simulink library "lib_affectiveChar_behavior"  (R2014a)
settings: Solver=ode45  StartTime=0.0  StopTime=10.0  RelTol=1e-3
libraries: simulink x5
(part 4 of 4)

== stateflow chart lib_affectiveChar_behavior/idlePoseRachel ==
  note: The higher BOREDOMT (treshold), the lower chance of bored pose.
  state stateRandomPose
    entry: interest=BOREDOM_THRESHOLD-boredom;
    entry: randPoseChance=randi([1,interest]);
  state sendBML(arg) [function]
  note: num of bmlID=18
  state stateBoredPose
    entry:
    sendBML( idlePoseRachelTable(randi([1,18])) );
  (default) -> stateRandomPose
  stateBoredPose -> stateRandomPose : after(1,secs)
  stateRandomPose -> (junction 2)
  (junction 2) -> stateRandomPose [order 2] : [randPoseChance~=1]
  (junction 2) -> stateRandomPose [order 3] : [isPosing~=0]
  (junction 2) -> stateBoredPose [order 1] : [([randPoseChance==1])&([isPosing==0])]
  data: arg function_input double size=[256 1]; bmlID function_input double; poseBML function_output double size=[256,1]; boredom data_store_memory size=2; BOREDOM_THRESHOLD data_store_memory size=2; randPoseChance data_store_memory size=2; isPosing data_store_memory size=2; interest data_store_memory size=2
  events: secs input RISING_EDGE_EVENT
  function poseBML=idlePoseRachelTable(bmlID):
    | function poseBML=idlePoseRachelTable(bmlID)
    | 
    | aVarTruthTableCondition_1 = false;
    | aVarTruthTableCondition_2 = false;
    | aVarTruthTableCondition_3 = false;
    | aVarTruthTableCondition_4 = false;
    | aVarTruthTableCondition_5 = false;
    | aVarTruthTableCondition_6 = false;
    | aVarTruthTableCondition_7 = false;
    | aVarTruthTableCondition_8 = false;
    | aVarTruthTableCondition_9 = false;
    | aVarTruthTableCondition_10 = false;
    | aVarTruthTableCondition_11 = false;
    | aVarTruthTableCondition_12 = false;
    | aVarTruthTableCondition_13 = false;
    | aVarTruthTableCondition_14 = false;
    | aVarTruthTableCondition_15 = false;
    | aVarTruthTableCondition_16 = false;
    | aVarTruthTableCondition_17 = false;
    | aVarTruthTableCondition_18 = false;
    | 
    | 
    | 
    | aVarTruthTableCondition_1 = logical(bmlID==1);
    | 
    | 
    | aVarTruthTableCondition_2 = logical(bmlID==2);
    | 
    | 
    | aVarTruthTableCondition_3 = logical(bmlID==3);
    | 
    | 
    | aVarTruthTableCondition_4 = logical(bmlID==4);
    | 
    | 
    | aVarTruthTableCondition_5 = logical(bmlID==5);
    | 
    | 
    | aVarTruthTableCondition_6 = logical(bmlID==6);
    | 
    | 
    | aVarTruthTableCondition_7 = logical(bmlID==7);
    | 
    | 
    | aVarTruthTableCondition_8 = logical(bmlID==8);
    | 
    | 
    | aVarTruthTableCondition_9 = logical(bmlID==9);
    | 
    | 
    | aVarTruthTableCondition_10 = logical(bmlID==10);
    | 
    | 
    | aVarTruthTableCondition_11 = logical(bmlID==11);
    | 
    | 
    | aVarTruthTableCondition_12 = logical(bmlID==12);
    | 
    | 
    | aVarTruthTableCondition_13 = logical(bmlID==13);
    | 
    | 
    | aVarTruthTableCondition_14 = logical(bmlID==14);
    | 
    | 
    | aVarTruthTableCondition_15 = logical(bmlID==15);
    | 
    | 
    | aVarTruthTableCondition_16 = logical(bmlID==16);
    | 
    | 
    | aVarTruthTableCondition_17 = logical(bmlID==17);
    | 
    | 
    | aVarTruthTableCondition_18 = logical(bmlID==18);
    | 
    | if (aVarTruthTableCondition_1)
    |     aFcnTruthTableAction_6();
    | elseif (aVarTruthTableCondition_2)
    |     aFcnTruthTableAction_2();
    | elseif (aVarTruthTableCondition_3)
    |     aFcnTruthTableAction_1();
    | elseif (aVarTruthTableCondition_4)
    |     aFcnTruthTableAction_2();
    | elseif (aVarTruthTableCondition_5)
    |     aFcnTruthTableAction_3();
    | elseif (aVarTruthTableCondition_6)
    |     aFcnTruthTableAction_7();
    | elseif (aVarTruthTableCondition_7)
    |     aFcnTruthTableAction_1();
    | elseif (aVarTruthTableCondition_8)
    |     aFcnTruthTableAction_3();
    | elseif (aVarTruthTableCondition_9)
    |     aFcnTruthTableAction_1();
    | elseif (aVarTruthTableCondition_10)
    |     aFcnTruthTableAction_6();
    | elseif (aVarTruthTableCondition_11)
    |     aFcnTruthTableAction_7();
    | elseif (aVarTruthTableCondition_12)
    |     aFcnTruthTableAction_5();
    | elseif (aVarTruthTableCondition_13)
    |     aFcnTruthTableAction_5();
    | elseif (aVarTruthTableCondition_14)
    |     aFcnTruthTableAction_3();
    | elseif (aVarTruthTableCondition_15)
    |     aFcnTruthTableAction_4();
    | elseif (aVarTruthTableCondition_16)
    |     aFcnTruthTableAction_3();
    | elseif (aVarTruthTableCondition_17)
    |     aFcnTruthTableAction_5();
    | elseif (aVarTruthTableCondition_18)
    |     aFcnTruthTableAction_5();
    | else % Default
    |     aFcnTruthTableAction_1();
    | end
    | 
    | function aFcnTruthTableAction_1()
    | 
    | % WeightShift
    | 
    | poseBML=encStr2Arr('<?xml version="1.0" ?><act><bml><animation name="ChrBrad@Idle01_WeightShift01" ready="1" relax="6" start="0" stroke="3 end="7"/></bml></act>');
    | 
    | function aFcnTruthTableAction_2()
    | 
    | % ScratchChest
    | 
    | poseBML=encStr2Arr('<?xml version="1.0" ?><act><bml><animation name="ChrRachel_ChrBrad@Idle01_ScratchChest01" /></bml></act>');
    | 
    | function aFcnTruthTableAction_3()
    | 
    | % ScratchHead
    | 
    | poseBML=encStr2Arr('<?xml version="1.0" ?><act><bml><animation name="ChrBrad@Idle01_ScratchHeadLf01" /></bml></act>');
    | 
    | function aFcnTruthTableAction_4()
    | 
    | % ShoulderStretchUpDown
    | 
    | poseBML=encStr2Arr('<?xml version="1.0" ?><act><bml><animation name="ChrBrad@Idle01_ShoulderStretch01" /></bml></act>');
    | 
    | function aFcnTruthTableAction_5()
    | 
    | % SqueezeHand01
    | 
    | poseBML=encStr2Arr('<?xml version="1.0" ?><act><bml><animation name="ChrBrad@Idle01_SqueezeHand01" /></bml></act>');
    | 
    | function aFcnTruthTableAction_6()
    | 
    | % WeightShift2
    | 
    | poseBML=encStr2Arr('<?xml version="1.0" ?><act><bml><animation name="ChrBrad@Idle01_WeightShift02" /></bml></act>');
    | 
    | function aFcnTruthTableAction_7()
    | 
    | % Idle01_ToIdle02
    | 
    | poseBML=encStr2Arr('<?xml version="1.0" ?><act><bml><animation name="ChrBrad@Idle01_ToIdle02" ready="1" relax="4" start="0" stroke="3" end="7"/></bml></act>');

== stateflow chart lib_affectiveChar_behavior/notImitateSmile ==
  state subSmile [parallel]
    settings: executionOrder=1
    state stateInitial
      entry: avert=1; gameState=14;
      n=encStr2Arr(' ');bmlsM=[n n n n n];newBmlsM=[n n n n n];
    state stateCheckSmile
    state gazeCamera
      entry:  [P,BMLM]= smileTable(2) ;avert=0;
      newBmlsM=insertQueue(bmlsM,BMLM);
      bmlsM=newBmlsM;
    state wait
    state checkP
      entry:  [P,BMLM]=  smileTable(1) ;
      newBmlsM=insertQueue(bmlsM,BMLM);
      bmlsM=newBmlsM;
    (default) -> stateInitial
    stateInitial -> stateCheckSmile
    subSmile.wait -> stateCheckSmile : after(10,secs)
    stateCheckSmile -> stateCheckSmile [order 2]
    gazeCamera -> stateCheckSmile [order 2] : after(1,secs)[isSmiling~=1]
    stateCheckSmile -> gazeCamera [order 1] : [[isSmiling==1]&[ gameState~= STATE_GO]&[ gameState~= STATE_READY]]
    checkP -> subSmile.wait
    gazeCamera -> checkP [order 1] : after(1,secs)[isSmiling==1]
  note: SMILE_DUER=10 seceonds
  note: check if still isSmiling is true works as a buffer to remove the smiles that last ony 1 sec (system errors).
  state subFacial [parallel]
    settings: executionOrder=2
    state stateFacialExpression
      entry:[au,au_L]=setAU(internalE);
      eAmountF =set_eAmountFactor(internalE,personality);
      BMLl=cmdBML_AUmerg(au,eAmountF);
      newBmlsL=insertQueueLow(bmlsL,BMLl);
      bmlsL=newBmlsL;
      %fprintf('%1.1f',internalE);disp(decArr2Str(BMLl));
    state initial
      entry:
      au=[0,0,0,0,0,0];
      au_L=0;
    state wait
    state wait2
    (default) -> initial
    subFacial.wait -> stateFacialExpression [order 1] : [internalE~=6]
    initial -> subFacial.wait
    stateFacialExpression -> subFacial.wait [order 1] : [internalE==6]
    subFacial.wait -> subFacial.wait [order 2]
    wait2 -> stateFacialExpression : [emoChange==1]
    stateFacialExpression -> wait2 [order 2] : [emoChange==0]
  data: bmls function_input double size=[1000,5]; myBML function_input double size=[1000,1]; newBmls function_output double size=[1000,5]; bmls function_input double size=[1000,5]; myBML function_input double size=[1000,1]; newBmls function_output double size=[1000,5]; bmlID function_input double; p function_output double size=1; poseBML function_output double size=[1000,1]; bmlID function_input double; p function_output double size=1; poseBML function_output double size=[1000,1]; E function_input double size=1; AU function_output double size=[1,6]; L function_output double size=1; E function_input double size=1; eAmountFactor function_output double size=[1,6]; Pt function_input double size=1; smileN local double size=1; isSmiling input double size=1 =0; avert data_store_memory =0; gazing data_store_memory size=2; GAZE_WIN data_store_memory size=2; BML data_store_memory size=[256,1]; P data_store_memory; fileID local double size=1; gameState output double; STATE_GO data_store_memory; STATE_READY data_store_memory; STATE_BEFORE data_store_memory; newBmlsM local double size=[1000,5]; bmlsM data_store_memory size=[256,1]; BMLM local double size=[1000,1]; n local; personality input double size=1; internalE input double size=1; au local; eAmountF local; emoChange input boolean size=1; au_i local double size=1; au_L local double size=1; emoDisp local; bmlsL data_store_memory size=[256,1]; BMLl local double size=[1000,1]; newBmlsL local double size=[1000,5]
  events: secs input RISING_EDGE_EVENT
  function newBmls =insertQueue(bmls,myBML):
    | function newBmls =insertQueue(bmls,myBML)
    |     full=1;
    |     t=encStr2Arr(' ');
    |     newBmls=[t t t t t];
    |     for i = 1:5
    |         if (isequal(bmls(:,i),t))
    |             %add to end of the queue where its empty
    |             bmls(:,i)=myBML;
    |             full=0;
    |             break
    |         end
    |     end
    |     if(full~=0)
    |             %if queue full, shift all elements to left which removes the first one, then add to end
    |             bmls(:,1)= bmls(:,2);
    |             bmls(:,2)= bmls(:,3);
    |             bmls(:,3)= bmls(:,4);
    |             bmls(:,5)=myBML;
    |     end
    |     newBmls=bmls;
  function newBmls =insertQueueLow(bmls,myBML):
    | function newBmls =insertQueueLow(bmls,myBML)
    |     full=1;
    |     t=encStr2Arr(' ');
    |     newBmls=[t t t t t];
    |     for i = 1:5
    |         if (isequal(bmls(:,i),t))
    |             %add to end of the queue where its empty
    |             bmls(:,i)=myBML;
    |             full=0;
    |             break
    |         end
    |     end
    |     if(full~=0)
    |             %if queue full, shift all elements to left which removes the first one, then add to end
    |             bmls(:,1)= bmls(:,2);
    |             bmls(:,2)= bmls(:,3);
    |             bmls(:,3)= bmls(:,4);
    |             bmls(:,5)=myBML;
    |     end
    |     newBmls=bmls;
  function [p,poseBML] = smileTable(bmlID):
    | function [p,poseBML] = smileTable(bmlID)
    | 
    | aVarTruthTableCondition_1 = false;
    | aVarTruthTableCondition_2 = false;
    | 
    | 
    | % smile
    | 
    | aVarTruthTableCondition_1 = logical(bmlID==1);
    | 
    | % headN
    | 
    | aVarTruthTableCondition_2 = logical(bmlID==2);
    | 
    | if (aVarTruthTableCondition_1)
    |     aFcnTruthTableAction_1();
    | elseif (aVarTruthTableCondition_2)
    |     aFcnTruthTableAction_2();
    | else % Default
    |     aFcnTruthTableAction_1();
    | end
    | 
    | function aFcnTruthTableAction_1()
    | 
    | % smile
    | 
    | poseBML=encStr2Arr('<?xml version="1.0"?><act><bml><face amount="1" au="12" side="BOTH" start="0" stroke="2" relax="3" end="4" type="facs"/><face amount="0.3" au="6" side="BOTH" start="0" stroke="2" relax="3" end="4" type="facs"/></bml></act>');p=3;
    | 
    | function aFcnTruthTableAction_2()
    | 
    | % headNeutralBrow
    | 
    | poseBML=encStr2Arr('<?xml version="1.0" ?><act><bml><gaze target="gazeTarget" start="0" end="5" sbm:time-hint="1.5"/></bml></act>');p=3;
    | 
    | function aFcnTruthTableAction_3()
    | 
    | % smileBrow
    | 
    | poseBML=encStr2Arr('<?xml version="1.0"?><act><bml><face amount="0.1" au="1" side="BOTH" start="0" stroke="2" relax="4" end="6" type="facs"/><face amount="0.1" au="2" side="BOTH" start="0" stroke="2" relax="4" end="6" type="facs"/></bml></act>');p=3;
  function [p,poseBML] = facialExpr(bmlID):
    | function [p,poseBML] = facialExpr(bmlID)
    | 
    | aVarTruthTableCondition_1 = false;
    | aVarTruthTableCondition_2 = false;
    | 
    | 
    | % smile
    | 
    | aVarTruthTableCondition_1 = logical(bmlID==1);
    | 
    | % headN
    | 
    | aVarTruthTableCondition_2 = logical(bmlID==2);
    | 
    | if (aVarTruthTableCondition_1)
    |     aFcnTruthTableAction_1();
    | elseif (aVarTruthTableCondition_2)
    |     aFcnTruthTableAction_2();
    | else % Default
    |     aFcnTruthTableAction_1();
    | end
    | 
    | function aFcnTruthTableAction_1()
    | 
    | % smile
    | 
    | poseBML=encStr2Arr('<?xml version="1.0"?><act><bml><face amount="1" au="12" side="BOTH" start="0" stroke="10" relax="70" end="100" type="facs"/><face amount="0.3" au="6" side="BOTH" start="0" stroke="10" relax="70" end="100" type="facs"/></bml></act>');p=3;
    | 
    | function aFcnTruthTableAction_2()
    | 
    | % headNeutralBrow
    | 
    | poseBML=encStr2Arr('<?xml version="1.0" ?><act><bml><gaze target="gazeTarget" start="0" end="5" sbm:time-hint="1.5"/></bml></act>');p=3;
    | 
    | function aFcnTruthTableAction_3()
    | 
    | % smileBrow
    | 
    | poseBML=encStr2Arr('<?xml version="1.0"?><act><bml><face amount="0.1" au="1" side="BOTH" start="0" stroke="2" relax="4" end="6" type="facs"/><face amount="0.1" au="2" side="BOTH" start="0" stroke="2" relax="4" end="6" type="facs"/></bml></act>');p=3;
  function [AU,L]=setAU(E):
    | function [AU,L]=setAU(E)	
    | % 1	Inner Brow Raiser,% 2	Outer Brow Raiser, % 4	Brow Lowerer
    | % 5	Upper Lid Raiser,% 6	Cheek Raiser,% 7	Lid Tightener
    | % 8	Lips Toward Each Other,% 9	Nose Wrinkler,% 10	Upper Lip Raiser	
    | % 11	Nasolabial Deepener	% 12	Lip Corner Puller % 13	Sharp Lip Puller % 14	Dimpler	
    | % 15	Lip Corner Depressor % 16	Lower Lip Depressor % 17	Chin Raiser	mentalis
    | % 18	Lip Pucker	% 19	Tongue Show	% 20	Lip Stretcher % 21	Neck Tightener	platysma
    | % 22	Lip Funneler% 23	Lip Tightener% 24	Lip Pressor % 25	Lips Part	depressor
    | % 26	Jaw Drop,% 27	Mouth Stretch
    | % 43	Eyes Closed, % 44	Eyebrow Gatherer,% 45	Blink,% 46	Wink
    | %smartbody no 43,15,17,10 looks wierd,no 142
    |    AU=[0,0,0,0,0,0];L=0;
    |    % AU5(eyeOpen) for A+
    |    % AU1,4 for V-
    |    %AU12 for V+
    |     switch(E)
    |         case 1 %V- A-,bored (43)[1]
    |             AU=[1,2,45,0,0,0];L=3;%[1,1,0.35]
    |         
    |         case 2 %V- A-;sad %(1,2,4,10,15,17,43)[];can be [1,2,4,45,6,0]
    |             AU=[1,4,0,0,0,0];L=2;%[1,1,0,0,0,0]
    |         
    |         case 3 %V- A+,frust(2,1,14)[1],(-1,-2,4,7,14)[2], maybe(1,7)[0.7,0.7,0.5]
    |             AU=[1,2,4,5,6,0];L=5;%[1,1,1,0.5,0.5,0]
    |         
    |         case 4 %V- A+,fear(1,2,4,5,25=mouth)
    |             AU=[1,2,4,5,6,7];L=6; %[1,1,1,0.2,0.2]
    |         
    |         case 5%V+ A-,calm
    |             AU=[12,14,0,0,0,0];L=2;%[0.7,0.3,0,0,0,0]
    |         
    |         case 7%V+ A+,happy
    |             AU=[6,12,0,0,0,0];L=2;%[1,0.5,0,0,0,0]
    |         
    |         case 8%V+ A+,excited
    |             AU=[12,26,5,1,2,0];L=5;%[1,1,1,1,1,0]
    |         
    |         case 9%V- A+, angry
    |             AU=[2,4,5,7,45,0];L=5;%[0.5,1,0.2,0.2,0.2]
    |         
    |         otherwise
    |             %confusion (1,2,4,7)[1] %[1,1,1,0.2]
    |             %worried (1,2,4,5) [1,1,1,0.5]
    |             %angry(4,5,7,10,27)[], can be(2,4,5,7,45)[0.5,1,0.2,0.2,0.2]
    | 
    |             AU=[0,0,0,0,0,0];L=0;
    |             disp('error, setAU,emotion not listed');
    |     end  
    | %[1]Craig S.D. et al(2004)emotions during learning:the first steps tw affect sensitive
    | %[2]grafsgard J F () automatically recog facial indicator of frust
  function eAmountFactor =set_eAmountFactor(E,Pt):
    | function eAmountFactor =set_eAmountFactor(E,Pt)
    |     AU=[0,0,0,0,0,0];eAmountFactor=[0,0,0,0,0,0];pFactor=0.5;
    |     %Note: make sure you change values in all 4 personalities
    |     if(Pt==1)
    |         %HEHN
    |         if(E==1)  %bored
    |             eAmountFactor=[1,1,0.37,0,0,0];
    |         elseif(E==2) %sad
    |             eAmountFactor=[1,1,0,0,0,0];
    |         elseif(E==3) %frust
    |             eAmountFactor=[1,1,1,0.5,0.5,0];
    |         elseif(E==4) %fear
    |             eAmountFactor=[1,1,1,0.2,0.2,0];
    |         elseif(E==5)%sleepy
    |             eAmountFactor=[0.7,0.3,0,0,0,0];
    |         elseif(E==7)%happy
    |             eAmountFactor=[0.38,1,0,0,0,0];
    |         elseif(E==8)%excited
    |             eAmountFactor=[0.5,0.2,0.6,0.6,0.6,0];    
    |         else          
    |             eAmountFactor=[0,0,0,0,0,0];
    |             disp('error, set_eAmountFactor,emotion not listed');
    |         end
    |     
    |         %LEHN  
    |     elseif(Pt==2)
    |         if(E==1)  %bored
    |             eAmountFactor=[1,1,0.37,0,0,0];
    |         elseif(E==2) %sad
    |             eAmountFactor=[1,1,0,0,0,0];
    |         elseif(E==3) %frust
    |             eAmountFactor=[1,1,1,0.5,0.5,0];
    |         elseif(E==4) %fear
    |             eAmountFactor=[1,1,1,0.2,0.2,0];
    |         elseif(E==5)%sleepy
    |             eAmountFactor=[0.7,0.3,0,0,0,0];
    |         elseif(E==7)%happy
    |             eAmountFactor=[0.38,1,0,0,0,0];
    |         elseif(E==8)%excited[12,26,5,1,2,0]
    |             eAmountFactor= [0.5,0.2,0.6,0.6,0.6,0];    
    |         else          
    |             eAmountFactor=[0,0,0,0,0,0];
    |             disp('error, set_eAmountFactor,emotion not listed');
    |         end
    | 
    |         %HELN
    |    elseif(Pt==3)
    |         if(E==1)  %bored
    |             eAmountFactor=[1,1,0.37,0,0,0];
    |         elseif(E==2) %sad
    |             eAmountFactor=[1,1,0,0,0,0];
    |         elseif(E==3) %frust
    |             eAmountFactor=[1,1,1,0.5,0.5,0];
    |         elseif(E==4) %fear
    |             eAmountFactor=[1,1,1,0.2,0.2,0];
    |         elseif(E==5)%sleepy
    |             eAmountFactor=[0.7,0.3,0,0,0,0];
    |         elseif(E==7)%happy
    |             eAmountFactor=[0.38,1,0,0,0,0];
    |         elseif(E==8)%excited[12,26,5,1,2,0]
    |             eAmountFactor=  [0.5,0.2,0.6,0.6,0.6,0];    
    |         else          
    |             eAmountFactor=[0,0,0,0,0,0];
    |             disp('error, set_eAmountFactor,emotion not listed');
    |         end
    |         eAmountFactor=eAmountFactor*pFactor;
    |         %LELN
    |     elseif(Pt==4)
    |         if(E==1)  %bored
    |             eAmountFactor=[1,1,0.37,0,0,0];
    |         elseif(E==2) %sad
    |             eAmountFactor=[1,1,0,0,0,0];
    |         elseif(E==3) %frust
    |             eAmountFactor=[1,1,1,0.5,0.5,0];
    |         elseif(E==4) %fear
    |             eAmountFactor=[1,1,1,0.2,0.2,0];
    |         elseif(E==5)%sleepy
    |             eAmountFactor=[0.7,0.3,0,0,0,0];
    |         elseif(E==7)%happy
    |             eAmountFactor=[0.38,1,0,0,0,0];
    |         elseif(E==8)%excited[12,26,5,1,2,0]
    |             eAmountFactor=  [0.5,0.2,0.6,0.6,0.6,0];    
    |         else          
    |             eAmountFactor=[0,0,0,0,0,0];
    |             disp('error, set_eAmountFactor,emotion not listed');
    |         end
    |         eAmountFactor=eAmountFactor*pFactor;
    |     end
    | %Following is if we want a same factor for each personaliy all through AUs
    | % function eAmountFactor =set_eAmountFactor(E,P)
    | %     AU=[6,12,142,0,0,0];eAMOUNT=[0,0,0,0,0,0];
    | %     switch E
    | %         case 1  %bored
    | %             eAMOUNT=[1,1,1,0,0,0];
    | %         case 2 %sad
    | %             eAMOUNT=[0.7,0.4,0.9,0,0,0];
    | %         case 3 %angry
    | %             eAMOUNT=[1,0.8,1,0,0,0];
    | %         case 4 %fear
    | %             eAMOUNT=[1,1,1,0,0,0];%5,6,7,26
    | %         case 5%contempt
    | %             eAMOUNT=[1,1,1,0,0,0];
    | %         case 7%happy
    | %             eAMOUNT=[0.2,1,0,0,0,0];
    | %         otherwise           
    | %             eAMOUNT=[0,0,0,0,0,0];
    | %             disp('error,amount for emotion not listed:');disp('eAMOUNT');
    | %     end 
    | %     switch P
    | %         case 1 %HEHN
    | %             pFactor=1;
    | %         case 2 %LEHN
    | %             pFactor=1;
    | %         case 3 %HELN
    | %             pFactor=0.5;
    | %         case 4 %LELN
    | %             pFactor=0.5;
    | %     end
    | %     eAmountFactor=pFactor*eAMOUNT;

== stateflow chart lib_affectiveChar_behavior/priorityCheck1 ==
  state init
  state checkP3
  state checkP1
  state checkP2
  state sendBML(BML)
  sendBML(BML) -> init : after(1,sec){flag=0;}
  init -> sendBML(BML) [order 1] : [priority==1]{flag=1;}
  init -> checkP1 [order 2] : [priority==2]
  checkP1 -> init [order 2] : [flag==1]
  init -> checkP3 [order 3] : [priority==3]
  checkP3 -> init [order 1] : [flag==1]
  checkP2 -> init [order 2] : [flag==2]
  checkP3 -> checkP2 [order 2]
  checkP1 -> sendBML(BML) [order 1] : [flag==0]{flag==2}
  checkP2 -> sendBML(BML) [order 1]

== stateflow chart lib_affectiveChar_behavior/Gaze/createGazePawn ==
  state sendSBM(arg) [function]
  state sendBML(arg) [function]
  state stateCreatePawn
    entry:
    sendSBM( encStr2Arr( 'gt = scene.createPawn("gazeTarget")' ) );
    sendBML(encStr2Arr('<?xml version="1.0" ?><act><bml><gaze sbm:joint-range="EYES BACK" target="gazeTarget"/></bml></act>'));
  (default) -> stateCreatePawn
  data: arg function_input double size=[256 1]; arg function_input double size=[256 1]

== matlab function lib_affectiveChar_behavior/Gaze/gazeControl/movePawn ==
  data: x input; y input; arrBML output
function arrBML   = fcn( x,y )
coder.extrinsic('sprintf')
%for agent to gaze at the user, we create a pawn where user stands and agent gazes at the pawn
%1) AnTS: x btw 200,600/gaze btw 0,1
 x=(x-200)/600;
c = countDigits(x);

mystr=blanks(66+c);
%mystr = sprintf('scene.getPawn(\"gazeTarget\").setPosition(SrVec(%d, %d ,%d))',x,0,150);
mystr = sprintf('scene.getPawn(\"gazeTarget\").setPosition(SrVec(%0.1f , %d ,%d))',x,1.7,2); %x btw 0,1
arrBML = encStr2Arr(mystr);

end

== stateflow chart lib_affectiveChar_behavior/priorityCheck ==
  state init
  state checkP3
  state checkP1
  state checkP2
  state sendBML(arg)
  sendBML(arg) -> init : after(1,sec){flag=0;}
  init -> sendBML(arg) [order 1] : [priority==1]{flag=1;}
  init -> checkP1 [order 2] : [priority==2]
  checkP1 -> init [order 2] : [flag==1]
  init -> checkP3 [order 3] : [priority==3]
  checkP3 -> init [order 1] : [flag==1]
  checkP2 -> init [order 2] : [flag==2]
  checkP3 -> checkP2 [order 2]
  checkP1 -> sendBML(arg) [order 1] : [flag==0]{flag==2}
  checkP2 -> sendBML(arg) [order 1]

== matlab function lib_affectiveChar_behavior/sharedFunc ==
  data: v function_input double size=1; a function_input double size=1; mutDurFactor function_output double size=1; avertDurFactor function_output double size=1; avertHeadFreqFactor function_output double size=1; p function_input double size=1; pFlag function_input boolean size=1; vaFlag function_input boolean size=1; avertHeadSpeed function_output double size=1; gazeArr function_input double size=[1,6]; avertDirsChance function_output double size=1; avertFreqFactor function_output double size=1; mutFreqFactor function_output double size=1; blinkFlag function_output double size=1; blinkPeriodMin function_output double size=1; blinkPeriodMax function_output double size=1; personalityChange function_input double size=1; headMutChance function_output double size=1; avertHeadDurFactor function_output double size=1; poseTwitch function_output double size=1; poseFreqFactor function_output double size=1; poseChanceFactor function_output double size=1; poseCatChance function_output double size=1; poseLean function_output double size=1; v function_input double size=1; ar function_input double size=1; p function_input double size=1; pFlag function_input boolean size=1; vaFlag function_input boolean size=1; poseSpeed function_output double size=1; poseSpace function_output double size=1; poseArr function_input double size=[1,6]; poseLeanFlag function_output double size=1; personalityChange function_input double size=1
function [mutDurFactor,avertDurFactor,avertHeadFreqFactor,avertHeadSpeed,avertDirsChance,avertFreqFactor,mutFreqFactor,blinkFlag,blinkPeriodMin,blinkPeriodMax,headMutChance,avertHeadDurFactor] =setGazeFactors(v,a,p,pFlag,vaFlag,gazeArr,personalityChange)
    % Valence/Arousal: ref?
    %V+A+ (excite,happy):high mutual dur,head avert freq less,high freq of change btw mut/avert(MMMMMMMAAMMMMMAMMMA)
    %V-A+ (fear,frust): mid mut/avert,,head avert freq mid,high freq of change btw mut/avert(MMAAMMMAAMMAAAMMMAAAMA)
    %V+A- (idle, calm): mid mut/avert,head avert freq mid,low freq of change btw mut/avert(MMMMMMMAAAAAAMMMMMAAAAA)
    %V-A- (bored,sad):  avert dur more,,head avert freq more,,high freq of change btw mut/avert(AAAAAAMAAAAAAAAMAAAAA)
    %V+A+: v>0 & a>0,V-A+: v<0 & a>0,V+A-:v>0 & a<0,V-A-:v<0 & a<0

    %paper: Effects of Direct and Averted Gaze on the Perception of Facially Communicated Emotion
    % rate of approach-oriented dispositions (i.e., anger and joy) higher for direct relative gaze stimuli
    %avoidance-oriented dispositions (i.e., fear and sadness) would be higher for averted gaze faces.

    %russel, mehrabian circumplex:
    % v-mid,a-mid:approach;     v-mid,a+:avoid;       v-mid,a-:avoid
    % v+,a-mid:mid-approach;    v+,a+:high-approach;  v+,a-:low-approach
    % v-,a-mid:mid-avoid;        v-,a+:high-avoid;    v-,a-:low-avoid

    % marsella, emotional gaze:
    % a+:high blink, faster move
    
    %PERSONALITY:
    % HEHN:mutual dur more,head avert freq more,high freq of change btw mut/avert(MAMAMMAMMMAMAMMAMMAMA)
    % LEHN:avert dur  more,head avert freq more, high freq of change btw mut/avert(AMAAMAAAMAMAAAMAAMAAM)
    % HELN:mutual dur  more,head avert freq less,low freq of change btw mut/avert(MMMMMMMAMMMMMMMMAMMM)
    % LELN:avert  dur more,head avert freq more,low freq of change btw mut/avert(AAAAAAMAAAAAAAAMAAAAA)
    
    %Perception of personality through eye gaze, Ruhland et al
    %Extravert: gaze tward,long,often,up-center-left-right; few blinks ; wide fast node
    %Introvert: gaze Avoidance,short,seldom,down-center; normal blinks; small slow node
    %Neurotic: gaze Avoidance,short,seldom,down-left-right; often blinks; None
    %Stable: gaze tward,medium,medium,center-left-right; normal blinks ; None
    
    %Saccadic reaction time is between 0.18sec and 0.22sec on average.Minimum intersaccadic interval ranges from 0.05sec to 0.1sec
    %smartbody DOF:magnitude:~btw 5'&12'->chanceO:btw 3&8->aveDur:btw 0.26sec&0.18sec --> 
    %simulation sample time is 0.001 so btw 26 and 18
    %magnitude=-6.9*log(chanceO/15.7) -->  -6.9*log(3/15.7)=11.4,-6.9*log(8/15.7)=4.6
    %chanceO=randArray(:,7)-->(3,8); 
    %avertDur=(25+2.5*magnitude)/2*factor;(same for mutual):btw(25+2.5*11.4)/2=26,(25+2.5*4.6)/2=18
    %randHeadChance=randi([1,1+round(randArray(3,5)/avert_head_frequency_factor)]);

    mutDurFactor=1; 
    avertDurFactor=1;  
    avertHeadDurFactor=1;
    avertHeadFreqFactor=30;
    avertHeadSpeed=1;%1=normal, 2=fast&up,3=slow&down
    avertDirsChance=0;%not 1 & 2 is normal
    avertFreqFactor=1;
    mutFreqFactor=1;
    blinkFlag=0;
    blinkPeriodMin=5.0; %normal
    blinkPeriodMax=9.0;%normal
    headMutChance=60;

    if(pFlag==1)
        if(personalityChange==1)
            blinkFlag=1;disp('personality changed.');
        end
        if(p==1)%HEHN  
            mutDurFactor=2; % HEHN mut longer ,12' to 17'((25+2.5*magnitude)*mutual_gaze_duration_factor)/7;
            avertDurFactor=0.5;%HE avert short,3' to 4',btw (25+2.5*magnitude)*avert_gaze_duration_factor)/7;
            
            mutFreqFactor=4;%HE mut alot
            avertFreqFactor=0.1;% HE avert gaze low
            
            avertHeadDurFactor=0.5;
            headMutChance=90;
            avertHeadFreqFactor=50;%HE often head,[avert_head_frequency_factor>randrandi(0,100)]
            avertHeadSpeed=2;%HE fast&up, headSpeed={1,2,3}
            avertDirsChance=1;%HE up            
            
            blinkPeriodMin=0.1; %HN often blinks
            blinkPeriodMax=2;%HE few blinks
            
        elseif(p==2) %LEHN %LE normal blinks, HN often blinks
            mutDurFactor=0.5; % LE mut less(mutDur/10) ,HN freq more
            avertDurFactor=2; % (avertDur/4)
            
            mutFreqFactor=0.1;
            avertFreqFactor=4;
            
            avertHeadDurFactor=2;%LEHN, HN change head a lot so not so high
            headMutChance=10;
            avertHeadFreqFactor=30;%LE avert low
            avertHeadSpeed=3;%LE slow&down
            avertDirsChance=2;%LE down
           
            blinkPeriodMin=0.1; %often
            blinkPeriodMax=3.0;%norm
        elseif(p==3) %HELN %HE few blinks, LN normal blinks 
            mutDurFactor=3; % HE dur more, LN freq less
            avertDurFactor=0.25;
            
            mutFreqFactor=4;
            avertFreqFactor=0.1;
            
            avertHeadDurFactor=0.25;%HE
            headMutChance=90;
            avertHeadFreqFactor=50;%HE avert head more
            avertHeadSpeed=2;%fast&up
            avertDirsChance=1;%HE up            
            
            blinkPeriodMin=6.0; %normal
            blinkPeriodMax=15.0;%few
        else %LELN %LE normal blinks, LN normal blinks 
            mutDurFactor=0.25; 
            avertDurFactor=3;
           
            mutFreqFactor=0.1;
            avertFreqFactor=4;
            
            avertHeadDurFactor=3.5;%LE
            headMutChance=10;
            avertHeadFreqFactor=20;%LE avert head less
            avertHeadSpeed=3;%slow&down
            avertDirsChance=2;%LE down
          
            blinkPeriodMin=5.0; %normal
            blinkPeriodMax=9.0;%normal
        end  
    end
%    I removed this since it intefere with personality's effect on gaze
%     if(vaFlag==1)%if V and A first are in this range and then go to less than them they will be reinitiated at the top
%         if(v>40 && a>40)%V+A+,high-approach,mutual alot
%             mutDurFactor=mutDurFactor*2; % /2
%             avertDurFactor=round(avertDurFactor*0.5);  % /2
%             avertHeadFreqFactor=round(avertHeadFreqFactor/3);%high-approach:head not avert
%             %avertHeadSpeed=2;%aroused fast, removed ths since fast&up is
%             %together, also it makes it hard for evaluateion
%             
%             %27-12-2015- Best way to set the blink period is as a linear
%             %function of arousal amount
%             %      val/(1+((2-1)*(A/100)))
%             %in which val is BlinkMin or BlinkMax and A is arousal amount;
%             %this function sets the blinkPriodMin and max to half for twice
%             %blink in arousal=100 and to their default at arousal=1 sicne
%             %we need to re-calculate and send sbms continiously I avoided
%             %that for
%             % now, instead I only increase min and max when Arousal passes
%             % 50 threshold
%             blinkPeriodMin=blinkPeriodMin/1.5; %often
%             blinkPeriodMax=blinkPeriodMax/1.5;
%             blinkFlag=1;
%             disp(mutDurFactor);
%         elseif(v<-40 && a>40) %V-A+,high-avoid, avert alot
%             mutDurFactor=round(mutDurFactor*0.5); % /2
%             avertDurFactor=avertDurFactor*2; % /2
%             avertHeadFreqFactor=avertHeadFreqFactor+30;%high-avoid:head avert alot
%             %avertHeadSpeed=2;%fast
%             blinkPeriodMin=blinkPeriodMin/1.5; %often
%             blinkPeriodMax=blinkPeriodMax/1.5;
%             blinkFlag=1;
%         elseif(v>40 && a<-40) %V+A- ,low-approach, mutual most
%             mutDurFactor=round(mutDurFactor*1.5); %  /2
%             avertDurFactor=round(avertDurFactor*0.75); %/2
%             avertHeadFreqFactor=round(avertHeadFreqFactor/2);%approach:head not avert
%             %avertHeadSpeed=1;%slow&down
%             blinkFlag=0;
%         elseif(v<-40 && a<-40) %V-A-,  low-avoid, avert most
%             mutDurFactor=round(mutDurFactor*0.75); %/2
%             avertDurFactor=round(avertDurFactor*1.5);% /2
%             avertHeadFreqFactor=avertHeadFreqFactor+20;%avoid:head avert alot
%             %avertHeadSpeed=1;%slow&down, if he is extrovert we dont want
%             %him to look down even if low aroused
%             blinkFlag=0;
%         end  
%         
%     end

== matlab function lib_affectiveChar_behavior/sharedFunc ==
function [poseTwitch,poseFreqFactor,poseChanceFactor,poseCatChance,poseLean,poseSpeed,poseSpace,poseLeanFlag]=setPoseFactors(v,ar,p,pFlag,vaFlag,poseArr,personalityChange)   
    
    pose_custom_flag=poseArr(:,1);
    pose_chance_custom=poseArr(:,3);
    pose_selfAdaptor_chance_custom=poseArr(:,2);
    pose_frequency_custom=poseArr(:,4);
    pose_speed_custom=poseArr(:,5);
    pose_lean_custom=poseArr(:,6);

    poseCatChance=50;%defalut 50% chance of selfA or weightShift, due low num of weightShift
    poseChanceFactor=1;%if (not similar duration btw poses always)
    poseFreqFactor=30;
    poseSpeed=1;%1=normal;2=fast; 3=slow;
    poseLean=18;
    poseTwitch=0;
    poseLeanFlag=0;
    poseSpace=0;% normal people dont do spacious gestures

    if(pose_custom_flag==0)    
        if(pFlag==1)
            if(personalityChange==1)
                poseLeanFlag=1;
            end
            if(p==1) %HEHN
                 poseTwitch=1;%HN
                 poseFreqFactor=15;%HN more freq,after(pose_frequency_factor,secs)
                 poseLean=18;
                 poseChanceFactor=4;% HN high chance,randPoseChance=randi([0,round(interest*randSlowPose/pose_chance_factor)]);
                 poseCatChance=90;%HN high selfA,[randPR<=pose_selfAdaptor_chance_factor ]
                 poseSpeed=2;%HE fast
                 poseSpace=0;%HE
             elseif(p==2)%LEHN
                 poseTwitch=1;%HN
                 poseFreqFactor=20;%HN more freq but low speed
                 poseLean=19;
                 poseChanceFactor=4;%HN high chance
                 poseCatChance=10;%HN high:90% adaptor
                 poseSpeed=3;%LE slow
                 poseSpace=0;%LE
             elseif(p==3)%HELN
                 poseTwitch=0;%LN
                 poseFreqFactor=45;%LN low chance
                 poseLean=18;
                 poseChanceFactor=1;%LN low chance
                 poseCatChance=10;%  10% adapter
                 poseSpeed=2;%HE
                 poseSpace=1;%HE
             elseif(p==4)%LELN
                 poseTwitch=0;%LN
                 poseFreqFactor=50;%LE
                 poseLean=19;
                 poseChanceFactor=1;%LN low chance
                 poseCatChance=90;
                 poseSpeed=3;%LE
                 poseSpace=0;%LE
            else%no personality, its should not come here
                fprintf(' Error: the personality is not listed, back to normal, p=: '); fprintf('%0.0f',p);
                poseCatChance=70;
                poseChanceFactor=1;
                poseFreqFactor=40;
                poseSpeed=1;%1=normal;2=fast; 3=slow;
                poseLean=18;
                poseTwitch=0;
                poseLeanFlag=0;
                poseSpace=0;% normal people dont do spacious gestures
             end
        end
%     29-12-2015  I removed this since it intefere with personality's effect on pose
%     % marsella, emotional gaze:
%     % a+:faster move,body fw
%     if(vaFlag==1)
%         if( ar>50)%A+
%              poseSpeed=2;%high arouse fast move
%              poseLeanFlag=12;%high aroused lean fw
%         end
%         if(ar<-50)%A-
%              poseSpeed=3;%low arouse slow move
%              poseLeanFlag=11;%low aroused lean back
%         end
%     end 
    
    else%custom-flag==1
        poseFreqFactor=pose_frequency_custom;
        poseLean=pose_lean_custom;
        poseChanceFactor=pose_chance_custom;
        poseCatChance=pose_selfAdaptor_chance_custom;
        poseSpeed=pose_speed_custom;
    end
